simulink model "EnergyHub_V5_inf_buffer"  (R2024b)
settings: Solver=VariableStepAuto  StartTime=0  StopTime=31536000  MaxStep=1  RelTol=1e-3
values from neighbouring files (symbols this model uses):
  BatteryVNom = 51.2    [EdgeCases.m]    (also in MultipleModelTesting.m; setup_V3.m; setup_V5.m)
  ElectrolyserBoP = 80    [EdgeCases.m]    (also in setup_V3.m; setup_V5.m)
  ElectrolyserHoldTime = 25 * 60    (= 1500)    [EdgeCases.m]    (also in setup_V3.m; setup_V5.m)
  ElectrolyserHyFlow = 510    [EdgeCases.m]    (also in setup_V3.m; setup_V5.m)
  ElectrolyserPower = 2450    [EdgeCases.m]    (also in setup_V3.m = 2450/2:2450/2:2450*1.5; setup_V5.m)
  ElectrolyserRampDownTime = 30 * 60    (= 1800)    [EdgeCases.m]    (also in setup_V3.m; setup_V5.m)
  ElectrolyserRampUpTime = 10 * 60    (= 600)    [EdgeCases.m]    (also in setup_V3.m; setup_V5.m)
  ElectrolyserWarming = 260    [EdgeCases.m]    (also in setup_V3.m; setup_V5.m)
  ElectrolyserWarmingTime = 12 * 60    (= 720)    [EdgeCases.m]    (also in setup_V3.m; setup_V5.m)
  EMSElecStartHr = 14    [EdgeCases.m]    (also in setup_V3.m = 12:0.5:15; setup_V5.m)
  EMSElecStartSoC = 70    [EdgeCases.m]    (also in setup_V3.m = 70:5:80; setup_V5.m)
  EMSElecStopSoC = 65    [EdgeCases.m]    (also in setup_V3.m = 50:5:65; setup_V5.m)
  EMSFCSoCThresholds = [140, 150, 160, 170, 180]    [EdgeCases.m]    (also in setup_V3.m = [13, 14, 15, 16, 17]; setup_V5.m)
  EMSFCStartSoC = 15    [EdgeCases.m]    (also in MultipleModelTesting.m; setup_V3.m = 25; setup_V5.m)
  EMSFCStopSoC = 70    [EdgeCases.m]    (also in MultipleModelTesting.m; setup_V3.m = 90; setup_V5.m)
  EMSFCTimeThresholds = [113, 114, 115, 116, 117]    [EdgeCases.m]    (also in setup_V3.m = [40, 50, 60, 70, 80]; setup_V5.m)
  FuelCellAirBlower = 6.4*33.9    (= 216.96)    [EdgeCases.m]    (also in setup_V3.m; setup_V5.m)
  FuelCellBoP = 155    [EdgeCases.m]    (also in setup_V3.m; setup_V5.m)
  FuelCellHyFlow = 24    [EdgeCases.m]    (also in setup_V3.m = 31.7333333333; setup_V5.m)
  FuelCellPower = 2380    [EdgeCases.m]    (also in setup_V3.m = 1.2e3:300:1.8e3; setup_V5.m)
  FuelCellRampDown = 60    [EdgeCases.m]    (also in setup_V3.m; setup_V5.m)
  FuelCellRampTime1 = 40    [EdgeCases.m]    (also in setup_V3.m; setup_V5.m)
  FuelCellRampTime2 = 18*60    (= 1080)    [EdgeCases.m]    (also in setup_V3.m; setup_V5.m)
  FuelCellStartPower = 580    [EdgeCases.m]    (also in setup_V3.m; setup_V5.m)
  GridExtra = 0    [EdgeCases.m]    (also in setup_V3.m; setup_V5.m = 50)
  HydrogenCapacity = 70    [EdgeCases.m]    (also in setup_V3.m = 48; setup_V5.m)
  MinSoCGrid = EMSFCStartSoC-5    (= 10)    [EdgeCases.m]    (also in MultipleModelTesting.m; setup_V5.m)
  SolarPanels = 21    [EdgeCases.m]    (also in MultipleModelTesting.m = 12; setup_V3.m = 12:3:18; setup_V5.m = 18)
  SummerBase = 80    [EdgeCases.m]    (also in setup_V3.m; setup_V5.m)
  WinterBase = 235    [EdgeCases.m]    (also in setup_V3.m; setup_V5.m)
undefined symbols (not defined in the file or in its folder): Ion, Lithium
libraries: spsACVoltageSourceLib x3, spsBatteryLib x1, spsControlledCurrentSourceLib x1, sps_lib x1, simulink x1, spsGroundLib x1, spsPower3phInstantaneousLib x1, spsThreePhaseDynamicLoadLib x1, spsThreePhaseVIMeasurementLib x1
(part 2 of 2)

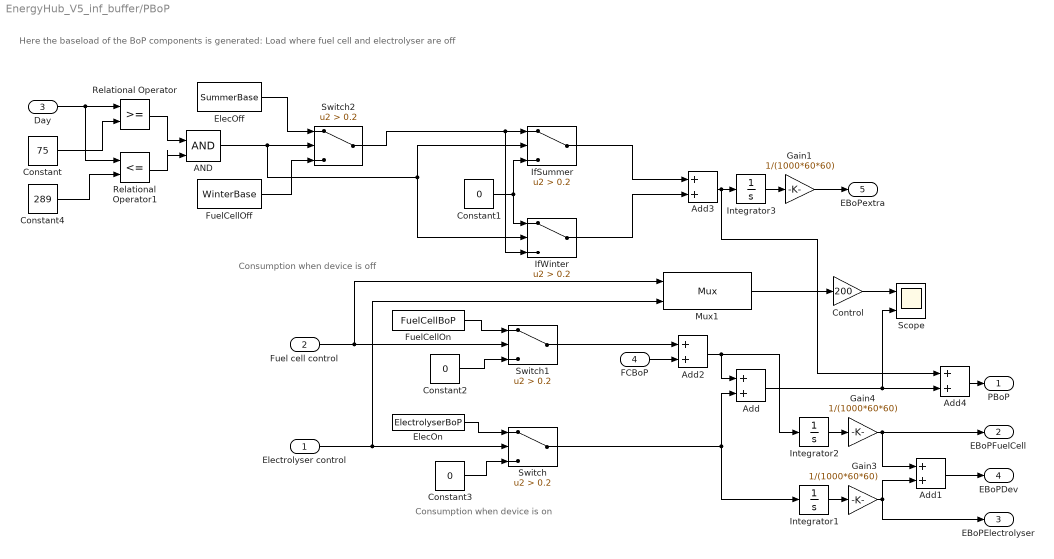
== system EnergyHub_V5_inf_buffer/PBoP ==
  note: Consumption when device is off
  note: Here the baseload of the
      | BoP components is generated:
      | Load where fuel cell and electrolyser are off
  note: Consumption when device is on
  Electrolyser control : Inport
  Fuel cell control : Inport  Port=2
  Day : Inport  Port=3
  FCBoP : Inport  Port=4
  AND : Logic  IconShape=distinctive  AllPortsSameDT=off  OutDataTypeStr=boolean
  Add{,1..4} (5 alike) : Sum
  Constant : Constant  Value=75
  Constant1 : Constant  Value=0
  Constant2 : Constant  Value=0
  Constant3 : Constant  Value=0
  Constant4 : Constant  Value=289
  Control : Gain  Gain=200
  ElecOff : Constant  Value=SummerBase
  ElecOn : Constant  Value=ElectrolyserBoP
  FuelCellOff : Constant  Value=WinterBase
  FuelCellOn : Constant  Value=FuelCellBoP
  Gain1 : Gain  Gain=1/(1000*60*60)
  Gain3 : Gain  Gain=1/(1000*60*60)
  Gain4 : Gain  Gain=1/(1000*60*60)
  IfSummer : Switch  Criteria=u2 > Threshold  Threshold=0.2  SaturateOnIntegerOverflow=off  InputSameDT=off
  IfWinter : Switch  Criteria=u2 > Threshold  Threshold=0.2  SaturateOnIntegerOverflow=off  InputSameDT=off
  Integrator1 : Integrator
  Integrator2 : Integrator
  Integrator3 : Integrator
  Mux1 : Mux  Inputs=2
      settings: DisplayOption=signals
  Relational Operator : RelationalOperator  OutDataTypeStr=boolean  RndMeth=Simplest  InputSameDT=off
  Relational Operator1 : RelationalOperator  Operator=<=  OutDataTypeStr=boolean  RndMeth=Simplest  InputSameDT=off
  Scope : Scope  NumInputPorts=2
  Switch : Switch  Criteria=u2 > Threshold  Threshold=0.2  SaturateOnIntegerOverflow=off  InputSameDT=off
  Switch1 : Switch  Criteria=u2 > Threshold  Threshold=0.2  SaturateOnIntegerOverflow=off  InputSameDT=off
  Switch2 : Switch  Criteria=u2 > Threshold  Threshold=0.2  SaturateOnIntegerOverflow=off  InputSameDT=off
  PBoP : Outport
  EBoPFuelCell : Outport  Port=2
  EBoPElectrolyser : Outport  Port=3
  EBoPDev : Outport  Port=4
  EBoPextra : Outport  Port=5
  wires:
  Switch/1 -> Add/2, Integrator1/1
  Add/1 -> Add4/2, Scope/2
  Add1/1 -> EBoPDev/1
  Gain3/1 -> Add1/2, EBoPElectrolyser/1
  Integrator1/1 -> Gain3/1
  Gain4/1 -> Add1/1, EBoPFuelCell/1
  Integrator2/1 -> Gain4/1
  ElecOn/1 -> Switch/1
  Electrolyser control/1 -> Mux1/2, Switch/2
  Fuel cell control/1 -> Mux1/1, Switch1/2
  FuelCellOn/1 -> Switch1/1
  Day/1 -> Relational Operator1/1, Relational Operator/1
  Constant/1 -> Relational Operator/2
  Constant4/1 -> Relational Operator1/2
  Relational Operator/1 -> AND/1
  Relational Operator1/1 -> AND/2
  AND/1 -> IfSummer/2, IfWinter/2, Switch2/2
  ElecOff/1 -> Switch2/1
  FuelCellOff/1 -> Switch2/3
  Switch2/1 -> IfWinter/3, IfSummer/1
  Constant1/1 -> IfWinter/1, IfSummer/3
  Control/1 -> Scope/1
  Mux1/1 -> Control/1
  Switch1/1 -> Add2/1
  FCBoP/1 -> Add2/2
  Add2/1 -> Add/1, Integrator2/1
  Constant2/1 -> Switch1/3
  Constant3/1 -> Switch/3
  IfSummer/1 -> Add3/1
  IfWinter/1 -> Add3/2
  Add3/1 -> Add4/1, Integrator3/1
  Integrator3/1 -> Gain1/1
  Gain1/1 -> EBoPextra/1
  Add4/1 -> PBoP/1

== system EnergyHub_V5_inf_buffer/PV generation ==
  From Workspace1 : FromWorkspace  VariableName=GTIdays  SampleTime=60  Interpolate=off  OutputAfterFinalValue=Setting to zero
  Gain : Gain  Gain=1/(1000*60*60)
  Integrator : Integrator
  Match Hours : TransportDelay  DelayTime=3600  BufferSize=5120
  eff : Gain  Gain=0.203
  m2 : Gain  Gain=SolarPanels*1.134*1.762
  PVPower : Outport
  PVEnergy : Outport  Port=2
  wires:
  Integrator/1 -> Gain/1
  Gain/1 -> PVEnergy/1
  m2/1 -> eff/1
  eff/1 -> Integrator/1, PVPower/1
  From Workspace1/1 -> Match Hours/1
  Match Hours/1 -> m2/1

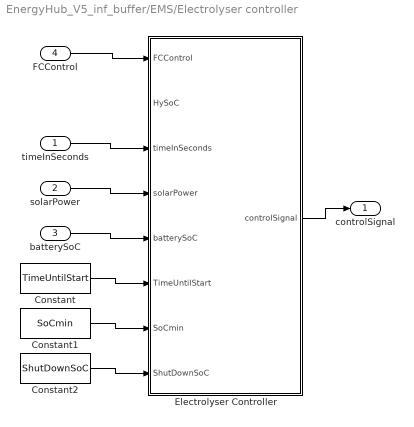
== system EnergyHub_V5_inf_buffer/EMS/Electrolyser controller ==
  timeInSeconds : Inport
  solarPower : Inport  Port=2
  batterySoC : Inport  Port=3
  FCControl : Inport  Port=4
  Constant : Constant  Value=TimeUntilStart
  Constant1 : Constant  Value=SoCmin
  Constant2 : Constant  Value=ShutDownSoC
  Electrolyser Controller : MATLAB Function  TreatAsAtomicUnit=on
  controlSignal : Outport
  wires:
  Electrolyser Controller/1(controlSignal) -> controlSignal/1
  batterySoC/1 -> Electrolyser Controller/5(batterySoC)
  timeInSeconds/1 -> Electrolyser Controller/3(timeInSeconds)
  solarPower/1 -> Electrolyser Controller/4(solarPower)
  Constant/1 -> Electrolyser Controller/6(TimeUntilStart)
  Constant1/1 -> Electrolyser Controller/7(SoCmin)
  Constant2/1 -> Electrolyser Controller/8(ShutDownSoC)
  FCControl/1 -> Electrolyser Controller/1(FCControl)

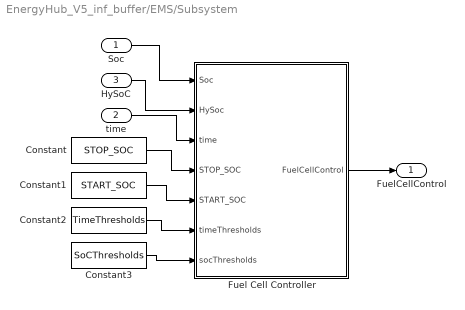
== system EnergyHub_V5_inf_buffer/EMS/Subsystem ==
  Soc : Inport
  time : Inport  Port=2
  HySoC : Inport  Port=3
  Constant : Constant  Value=STOP_SOC
  Constant1 : Constant  Value=START_SOC
  Constant2 : Constant  Value=TimeThresholds
  Constant3 : Constant  Value=SoCThresholds
  Fuel Cell Controller : MATLAB Function  TreatAsAtomicUnit=on
  FuelCellControl : Outport
  wires:
  Soc/1 -> Fuel Cell Controller/1(Soc)
  Fuel Cell Controller/1(FuelCellControl) -> FuelCellControl/1
  time/1 -> Fuel Cell Controller/3(time)
  Constant/1 -> Fuel Cell Controller/4(STOP_SOC)
  Constant1/1 -> Fuel Cell Controller/5(START_SOC)
  Constant3/1 -> Fuel Cell Controller/7(socThresholds)
  Constant2/1 -> Fuel Cell Controller/6(timeThresholds)
  HySoC/1 -> Fuel Cell Controller/2(HySoc)

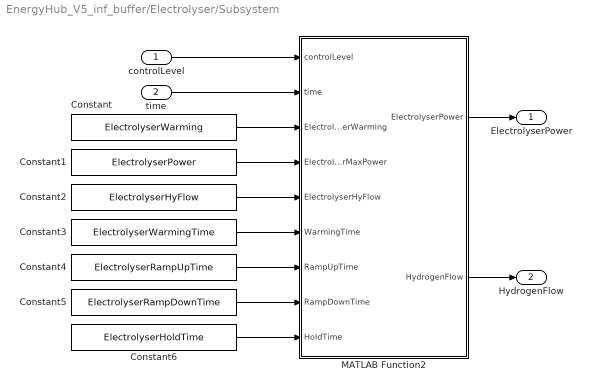
== system EnergyHub_V5_inf_buffer/Electrolyser/Subsystem ==
  controlLevel : Inport
  time : Inport  Port=2
  Constant : Constant  Value=ElectrolyserWarming
  Constant1 : Constant  Value=ElectrolyserPower
  Constant2 : Constant  Value=ElectrolyserHyFlow
  Constant3 : Constant  Value=ElectrolyserWarmingTime
  Constant4 : Constant  Value=ElectrolyserRampUpTime
  Constant5 : Constant  Value=ElectrolyserRampDownTime
  Constant6 : Constant  Value=ElectrolyserHoldTime
  MATLAB Function2 : MATLAB Function  TreatAsAtomicUnit=on
  ElectrolyserPower : Outport
  HydrogenFlow : Outport  Port=2
  wires:
  MATLAB Function2/2(HydrogenFlow) -> HydrogenFlow/1
  MATLAB Function2/1(ElectrolyserPower) -> ElectrolyserPower/1
  controlLevel/1 -> MATLAB Function2/1(controlLevel)
  time/1 -> MATLAB Function2/2(time)
  Constant/1 -> MATLAB Function2/3(ElectrolyserWarming)
  Constant1/1 -> MATLAB Function2/4(ElectrolyserMaxPower)
  Constant2/1 -> MATLAB Function2/5(ElectrolyserHyFlow)
  Constant3/1 -> MATLAB Function2/6(WarmingTime)
  Constant4/1 -> MATLAB Function2/7(RampUpTime)
  Constant5/1 -> MATLAB Function2/8(RampDownTime)
  Constant6/1 -> MATLAB Function2/9(HoldTime)

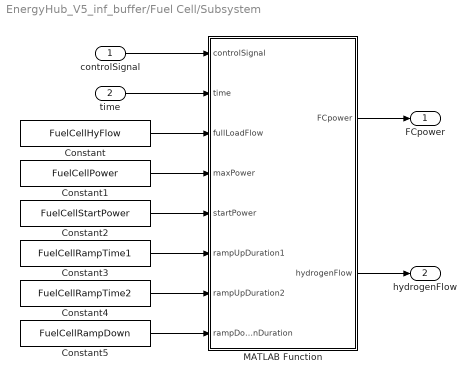
== system EnergyHub_V5_inf_buffer/Fuel Cell/Subsystem ==
  controlSignal : Inport
  time : Inport  Port=2
  Constant : Constant  Value=FuelCellHyFlow
  Constant1 : Constant  Value=FuelCellPower
  Constant2 : Constant  Value=FuelCellStartPower
  Constant3 : Constant  Value=FuelCellRampTime1
  Constant4 : Constant  Value=FuelCellRampTime2
  Constant5 : Constant  Value=FuelCellRampDown
  MATLAB Function : MATLAB Function  TreatAsAtomicUnit=on
  FCpower : Outport
  hydrogenFlow : Outport  Port=2
  wires:
  MATLAB Function/2(hydrogenFlow) -> hydrogenFlow/1
  controlSignal/1 -> MATLAB Function/1(controlSignal)
  MATLAB Function/1(FCpower) -> FCpower/1
  time/1 -> MATLAB Function/2(time)
  Constant/1 -> MATLAB Function/3(fullLoadFlow)
  Constant2/1 -> MATLAB Function/5(startPower)
  Constant1/1 -> MATLAB Function/4(maxPower)
  Constant3/1 -> MATLAB Function/6(rampUpDuration1)
  Constant4/1 -> MATLAB Function/7(rampUpDuration2)
  Constant5/1 -> MATLAB Function/8(rampDownDuration)

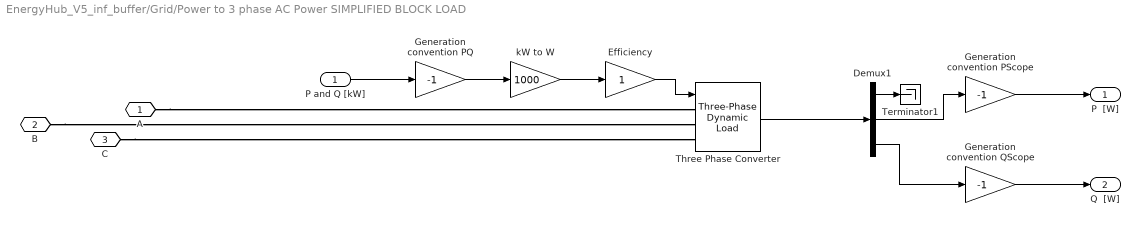
== system EnergyHub_V5_inf_buffer/Grid/Power to 3 phase AC Power SIMPLIFIED BLOCK LOAD ==
  P and Q [kW] : Inport
  Demux1 : Demux  Outputs=3
      settings: DisplayOption=none
  Efficiency : Gain
  Generation convention PQ : Gain  Gain=-1
  Generation convention PScope : Gain  Gain=-1
  Generation convention QScope : Gain  Gain=-1
  Terminator1 : Terminator
  Three Phase Converter : spsThreePhaseDynamicLoadLib/Three-Phase Dynamic Load  NominalVoltage=[ 400 50 ]  ActiveReactivePowers=[50e+003 0]  PositiveSequence=[0.98441 -1.41063]  ExternalControl=on  NpNq="[1  1]"  TimeConstants="[0  0  0  0]"  MinimumVoltage=0.7  Tfilter=1e-4  LoadFlowParameters=[4 50000000 0 0 25000000]
  kW to W : Gain  Gain=1000
  A : PMIOPort  Side=Left
  B : PMIOPort  Port=2  Side=Left
  C : PMIOPort  Port=3  Side=Left
  "P  [W] " : Outport
  "Q  [W] " : Outport  Port=2
  wires:
  Demux1/1 -> Terminator1/1
  Efficiency/1 -> Three Phase Converter/1
  kW to W/1 -> Efficiency/1
  Generation convention PQ/1 -> kW to W/1
  P and Q [kW]/1 -> Generation convention PQ/1
  Generation convention PScope/1 -> "P  [W] "/1
  Demux1/2 -> Generation convention PScope/1
  Demux1/3 -> Generation convention QScope/1
  Generation convention QScope/1 -> "Q  [W] "/1
  Three Phase Converter/1 -> Demux1/1
  connections:
  A/RConn1 -- Three Phase Converter/LConn1
  C/RConn1 -- Three Phase Converter/LConn3
  B/RConn1 -- Three Phase Converter/LConn2

== matlab function EnergyHub_V5_inf_buffer/Electrolyser/Subsystem/MATLAB Function2 ==
  settings: updateMethod=DISCRETE
  data: controlLevel input; ElectrolyserPower output; time input; HydrogenFlow output; ElectrolyserWarming input; ElectrolyserMaxPower input; ElectrolyserHyFlow input; WarmingTime input; RampUpTime input; RampDownTime input; HoldTime input
function [ElectrolyserPower, HydrogenFlow] = Electrolyser(controlLevel, time, ElectrolyserWarming, ElectrolyserMaxPower, ElectrolyserHyFlow, WarmingTime, RampUpTime, RampDownTime, HoldTime)
    % Inputs:
    % controlLevel (double): Control level between 0.6 and 1.0, 0 means off, and values between 0.6 and 1.0 represent the operational level
    % time (double): Simulation time in seconds
    
    % Outputs:
    % ElectrolyserPower (double): Power consumed by the electrolyser
    % HydrogenFlow (double): Hydrogen flow rate
    
    % Constants
    %ElectrolyserWarming = 260;  % [W] Electrolyser Warming Power Consumption
    %ElectrolyserPower = 2450;   % [W] Electrolyser Max Power Consumption
    %ElectrolyserHyFlow = 510;
    %WarmingTime = 12 * 60; % 12 minutes in seconds
    %RampUpTime = 10 * 60; % 10 minutes in seconds
    %RampDownTime = 30 * 60;
    RampDownStartPower = 0.6 * ElectrolyserMaxPower;
    RampDownStartHy = 0.6 * ElectrolyserHyFlow;
    %HoldTime = 25 * 60;         % Time before electrolyser actually turns off after off signal

    % Logic for output control
    persistent startTime isRampActive stopTime isRampingDown currentPower currentHydrogen;

    % Initialize persistent variables
    if isempty(startTime) || isempty(isRampActive) || isempty(isRampingDown) || isempty(stopTime)
        startTime = NaN;
        stopTime = NaN;
        isRampActive = false;
        isRampingDown = false;
        currentPower = 0;
        currentHydrogen = 0;
    end

    % Default outputs
    ElectrolyserPower = 0;
    HydrogenFlow = 0;

    % Initialize target variables
    targetPower = 0;
    targetHydrogen = 0;

    % If the control level is nonzero (system is on)
    if controlLevel > 0
        % If the system has not started before, record the start time
        if isnan(startTime)
            startTime = time;
            isRampActive = false; % Start with constant output
        end

        % If the system has been running for 12 minutes, start ramping
        if (time - startTime) >= WarmingTime && ~isRampActive
            isRampActive = true; % Start ramping after 12 minutes
        end

        % If the system is ramping
        if isRampActive
            % Calculate elapsed time for ramp-up
            rampElapsedTime = time - startTime - WarmingTime;

            % If the ramping time has not yet completed, linearly ramp from 260 to 2450
            if rampElapsedTime <= RampUpTime
                targetPower = ElectrolyserWarming + (ElectrolyserMaxPower - ElectrolyserWarming) * (rampElapsedTime / RampUpTime) * controlLevel;
                targetHydrogen = 0 + (ElectrolyserHyFlow - 0) * (rampElapsedTime / RampUpTime) * controlLevel;
            else
                % Once ramp-up is complete, keep the output at the final ramp values scaled by controlLevel
                targetPower = ElectrolyserMaxPower * controlLevel;
                targetHydrogen = ElectrolyserHyFlow * controlLevel;
            end
        else
            % If still within the first 12 minutes, output the constant value scaled by controlLevel
            targetPower = ElectrolyserWarming; %* controlLevel;
            targetHydrogen = 0; % Assume no hydrogen flow during the constant phase
        end
    else
        % Check if the system was previously on before ramping down
        if ~isnan(startTime)
            if isnan(stopTime)
                stopTime = time; % Record time when system turned off
                isRampingDown = true;
            end

            rampDownElapsedTime = time - stopTime;

            if isRampingDown
                if rampDownElapsedTime <= RampDownTime
                    % Ramp down power from previous state
                    targetPower = currentPower - (currentPower - RampDownStartPower * controlLevel) * (rampDownElapsedTime / RampDownTime);
                    targetHydrogen = currentHydrogen - (currentHydrogen - RampDownStartHy * controlLevel) * (rampDownElapsedTime / RampDownTime);
                elseif rampDownElapsedTime <= (RampDownTime + HoldTime)
                    % Hold at 60% power
                    targetPower = RampDownStartPower * controlLevel;
                    targetHydrogen = RampDownStartHy * controlLevel;
                else
                    % Fully shut down
                    targetPower = 0;
                    targetHydrogen = 0;
                    isRampingDown = false; % Stop ramp-down process
                    startTime = NaN; % Fully reset system
                    stopTime = NaN;
                    isRampActive = false;
                end
            end
        else
            % If the system was never on, ensure it stays off
            targetPower = 0;
            targetHydrogen = 0;
        end
    end

    % Smooth transition to target values
    rampRate = 50; % Rate of power change per time step
    if currentPower < targetPower
        currentPower = min(currentPower + rampRate, targetPower);
    elseif currentPower > targetPower
        currentPower = max(currentPower - rampRate, targetPower);
    end

    if currentHydrogen < targetHydrogen
        currentHydrogen = min(currentHydrogen + rampRate, targetHydrogen);
    elseif currentHydrogen > targetHydrogen
        currentHydrogen = max(currentHydrogen - rampRate, targetHydrogen);
    end

    ElectrolyserPower = currentPower;
    HydrogenFlow = currentHydrogen;
end

== matlab function EnergyHub_V5_inf_buffer/EMS/Subsystem/Fuel Cell Controller ==
  settings: updateMethod=DISCRETE
  data: Soc input; HySoc input; time input; FuelCellControl output; STOP_SOC input; START_SOC input; timeThresholds input; socThresholds input
function FuelCellControl = fuelCellControl(Soc, HySoc, time,STOP_SOC, START_SOC, timeThresholds, socThresholds)
    % Inputs:
    % Soc: Battery State of Charge (SoC) in percentage (0-100)
    % time: Current simulation time in seconds
    
    % Outputs:
    % FuelCellControl: on (1) or off (0)
    
    % Constants
    % STOP_SOC, Stop fuel cell if SoC > 90%
    % START_SOC, Start fuel cell if SoC < 25%
    
    % Define SoC thresholds for different times of day
    % timeThresholds, 13:00, 14:00, 15:00, 16:00, 17:00 (in hours)
    % socThresholds, 40, 50, 60, 70, 80: Corresponding SoC thresholds
    
    % Convert time from seconds to hours
    timeInHours = mod(time / 3600, 24);
    
    % Persistent variable to track whether the fuel cell remains on
    persistent hasRunToday;  % Tracks whether the electrolyzer has run today
    persistent Remain;
    persistent lastDay;      % Tracks the last day for resetting logic
    persistent firstSimulatedDay;

    
    if isempty(Remain)
        Remain = 0;         % Initialize to off
    end
    
    if isempty(hasRunToday)
       hasRunToday = true;      % Initially, the electrolyzer has not run today
       lastDay = -2;            % Initialize to an invalid day number
    end
    % Convert time from seconds to hours and extract the hour of the day
    currentDay = floor(time / 86400);      % Day number (0, 1, 2, ...)
    secondsInDay = 86400;
    dayOfYear = floor(time / secondsInDay) + 1; % Day of the year (1 to 365/366)

    OperationalDaysStop = 75;       % Last day of normal fuel cell operation
    OperationalDaysStart = 289;     % First day of normal fuel cell operation

    % Check if the day has changed (midnight reset)
    if currentDay ~= lastDay
       hasRunToday = false;
       lastDay = currentDay; 
       disp(sprintf('New day: %d', int32(currentDay)));   % Prints the current day in the console to track progression
    end

    if isempty(firstSimulatedDay)
        firstSimulatedDay = floor(time / 86400);
    end

    % Ensure fuel cell is off only during the first night of the first simulated day
    if (currentDay == firstSimulatedDay) && (timeInHours < 13)
        FuelCellControl = 0;
        return;
    end

    FuelCellControl = 0; % Initially off


    % Logic to control the fuel cell
  
  
    if Soc < START_SOC
        FuelCellControl = 1;
        Remain = 1;
    elseif Soc > STOP_SOC
        FuelCellControl = 0;
        Remain = 0;
    elseif (Soc >= START_SOC && Soc <= STOP_SOC && currentDay ~= 0)
        if Remain == 1
            FuelCellControl = 1;                % Keep the fuel cell on
            hasRunToday = true;
        else
            for i = 1:length(timeThresholds)    % Check the conditions of the 
                if (timeInHours >= timeThresholds(i) && (i == length(timeThresholds) || timeInHours < timeThresholds(i+1))) && Soc < socThresholds(i) && ~hasRunToday && (dayOfYear <= OperationalDaysStop|| dayOfYear >= OperationalDaysStart )
                    FuelCellControl = 1;        % Fuel cell on
                    hasRunToday = true;
                    Remain = 1;                 % Update Remain to keep it on
                    break;
                end
            end
        end
    end
end

== matlab function EnergyHub_V5_inf_buffer/EMS/Electrolyser controller/Electrolyser Controller ==
  settings: updateMethod=DISCRETE
  data: FCControl input; HySoC input; timeInSeconds input; controlSignal output; solarPower input; batterySoC input; TimeUntilStart input; SoCmin input; ShutDownSoC input
function controlSignal = electrolyzerControl(FCControl, HySoC, timeInSeconds, solarPower, batterySoC, TimeUntilStart, SoCmin, ShutDownSoC)
    % Inputs:
    % - timeInSeconds: Current simulation time in seconds, to determine day
    % - solarPower: Solar power available in W
    % - batterySoC: Battery state of charge in % (0 to 100)
   
    % Output:
    % - controlSignal: 0 = OFF, 0.6 to 1.0 = ON

    % Persistent variables to store state across time steps
    persistent hasRunToday;         % Tracks whether the electrolyzer has run today
    persistent FCHasRunToday;       % Tracks whether the fuel cell has
    persistent FCHasRunYesterday;   % Tracks whether the fuel cell has run yesterday
    persistent lastDay;             % Tracks the last day for resetting logic
    persistent isElectrolyzerOn;    % Tracks whether the electrolyzer is on
    persistent currentControlLevel; % Tracks the current control level

    % Initialize persistent variables
    if isempty(hasRunToday)
        hasRunToday = false;     % Initially, the electrolyzer has not run today
        FCHasRunToday = false;   % Initially, the fuel cell has not run today
        FCHasRunYesterday = false; % Initially, the fuel cell has not run yesterday

        lastDay = -1;            % Initialize to an invalid day number
        isElectrolyzerOn = false; % Initially OFF
        
        currentControlLevel = 0;  % Initially OFF
    end

    % Convert time from seconds to hours and extract the hour of the day
    timeInHours = mod(timeInSeconds, 86400) / 3600; % Hours within a single day
    currentDay = floor(timeInSeconds / 86400);      % Day number (0, 1, 2, ...)

    % Check if the day has changed (midnight reset)
    if currentDay ~= lastDay
        hasRunToday = false;     % Reset for the new day
        FCHasRunYesterday = FCHasRunToday; % Yesterday's FC activity is stored
        FCHasRunToday = false;   % Reset FC run tracking
        lastDay = currentDay;    % Update the lastDay variable
    end

    if FCControl > 0
        FCHasRunToday = true;
    end


    % ON condition: Turn ON the electrolyzer if all conditions are met
    if ~isElectrolyzerOn && ~hasRunToday && batterySoC > SoCmin && solarPower > 1000 && timeInHours < TimeUntilStart && ~FCHasRunToday && ~FCHasRunYesterday
        isElectrolyzerOn = true;  % Turn ON the electrolyzer
        hasRunToday = true;       % Mark as run for the day
    end

    % OFF condition: Turn OFF the electrolyzer if any OFF condition is met
    if isElectrolyzerOn && (batterySoC < ShutDownSoC || solarPower < 50)
        isElectrolyzerOn = false; % electrolyser is shut off
    end

    % Set control signal based on battery SoC when ON
    if isElectrolyzerOn
        targetControlLevel = 0.6 + (batterySoC - SoCmin) / 10  * 0.4; % Scale between 0.6 and 1.0 for SoC ranges
        targetControlLevel = max(0.6, min(targetControlLevel, 1.0));  % Saturate output
        
        % Ramp-up behavior
        rampRate = 0.05; % Rate at which control level increases per step
        if currentControlLevel < targetControlLevel
            currentControlLevel = min(currentControlLevel + rampRate, targetControlLevel);
        elseif currentControlLevel > targetControlLevel
            currentControlLevel = max(currentControlLevel - rampRate, targetControlLevel);
        end
    else
        currentControlLevel = 0; % OFF state
    end
    controlSignal = currentControlLevel;
end

== matlab function EnergyHub_V5_inf_buffer/Fuel Cell/Subsystem/MATLAB Function ==
  settings: updateMethod=DISCRETE
  data: controlSignal input; FCpower output; time input; hydrogenFlow output; fullLoadFlow input; maxPower input; startPower input; rampUpDuration1 input; rampUpDuration2 input; rampDownDuration input
function [FCpower, hydrogenFlow] = fuelCell(controlSignal, time, fullLoadFlow, maxPower, startPower, rampUpDuration1, rampUpDuration2, rampDownDuration)
   % Define the ramp-up and ramp-down parameters
   %rampUpDuration1 = 40; % seconds to ramp from 0W to 500W
   % rampUpDuration2 = 18 * 60; % seconds to ramp from 500W to 1.83kW
   % startPower = 580;
   % maxPower = 1.83e3; % Maximum power in watts (1.83 kW)
    minPower = 0; % Minimum power (0W)
   % fullLoadFlow = 24; % Hydrogen flow rate at full load (NL/min)
   % rampDownDuration = 60; % seconds to ramp down from 1.83kW to 0W

    % Initialize output values
    FCpower = 0;
    hydrogenFlow = 0;

   persistent startTime stopTime isRampActive;
   % Initialize persistent variables
   if isempty(startTime) || isempty(isRampActive) || isempty(stopTime)
       startTime = NaN;
       stopTime = NaN;
       isRampActive = false;
   end
  
    % Check control signal (assuming high is 1 and low is 0)
    if controlSignal == 1       
        if isnan(startTime)
           startTime = time;
           isRampActive = false; % Start with constant output
        end

        rampElapsedTime = time - startTime;

        % Fuel cell is ON, calculate output power and hydrogen flow rate
        if rampElapsedTime <= rampUpDuration1
            % Ramp-up from 0W to 500W in 40 seconds
            FCpower = (startPower / rampUpDuration1) * rampElapsedTime;
        elseif rampElapsedTime <= (rampUpDuration1 + rampUpDuration2)
            % Ramp-up from 500W to 1.83kW in 15 minutes (900 seconds)
            timeInRampUp2 = rampElapsedTime - rampUpDuration1;
            FCpower = startPower + ((maxPower - startPower) / rampUpDuration2) * timeInRampUp2;
        elseif rampElapsedTime > (rampUpDuration1 + rampUpDuration2)
            % Keep the power at 1.83 kW
            FCpower = maxPower;
        end
        
        % Hydrogen flow rate follows the same pattern as power output
        hydrogenFlow = (fullLoadFlow / maxPower) * FCpower;
        
    elseif controlSignal == 0
        % Fuel cell is OFF, calculate ramp-down behavior
        if time <= rampDownDuration
            % Ramp-down from 1.83 kW to 0W in 1 minute
            FCpower = maxPower * (1 - (time / rampDownDuration));
        else
            % Fuel cell is completely off
            FCpower = 0;
            hydrogenFlow = 0;
            startTime = NaN;
        end
    end
end

== matlab function EnergyHub_V5_inf_buffer/Electrolyser/MATLAB Function1 ==
  settings: updateMethod=DISCRETE
  data: startSystem input; ElectrolyserPower output; time input; HydrogenFlow output
function [ElectrolyserPower, HydrogenFlow] = Electrolyser(startSystem, time)
    % Inputs:
    % startSystem (boolean): Indicates whether the system is allowed to start
    % time (double): Simulation time in seconds
    
    % Outputs:
    % ElectrolyserPower (double): Power consumed by the electrolyser
    % HydrogenFlow (double): Hydrogen flow rate
    
    % Constants
    CONSTANT_OUTPUT = 260;
    RAMP_OUTPUT_END = 2450;
    RAMP_OUTPUT_END2 = 510;
    CONSTANT_TIME = 12 * 60; % 12 minutes in seconds
    RAMP_TIME = 10 * 60; % 10 minutes in seconds
    RAMP_DOWN_TIME = 30 * 60;
    RAMP_DOWN_START = 0.6*RAMP_OUTPUT_END;
    RAMP_DOWN_START2 = 0.6* RAMP_OUTPUT_END2;
    HOLD_TIME = 25*60;

    % Logic for output control
    persistent startTime isRampActive stopTime isRampingDown;

    % Initialize persistent variables
    if isempty(startTime) || isempty(isRampActive) || isempty(isRampingDown) || isempty(stopTime)
        startTime = NaN;
        stopTime = NaN;
        isRampActive = false;
        isRampingDown = false;
    end

    % Default outputs
    ElectrolyserPower = 0;
    HydrogenFlow = 0;

    % If the system is turned on
    if startSystem
        % If the system has not started before, record the start time
        if isnan(startTime)
            startTime = time;
            isRampActive = false; % Start with constant output
        end

        % If the system has been running for 12 minutes, start ramping
        if (time - startTime) >= CONSTANT_TIME && ~isRampActive
            isRampActive = true; % Start ramping after 12 minutes
        end

        % If the system is ramping
        if isRampActive
            % Calculate elapsed time for ramp-up
            rampElapsedTime = time - startTime - CONSTANT_TIME;

            % If the ramping time has not yet completed, linearly ramp from 260 to 2450
            if rampElapsedTime <= RAMP_TIME
                ElectrolyserPower = CONSTANT_OUTPUT + (RAMP_OUTPUT_END - CONSTANT_OUTPUT) * (rampElapsedTime / RAMP_TIME);
                HydrogenFlow = 0 + (RAMP_OUTPUT_END2 - 0) * (rampElapsedTime / RAMP_TIME);
            else
                % Once ramp-up is complete, keep the output at the final ramp values
                ElectrolyserPower = RAMP_OUTPUT_END;
                HydrogenFlow = RAMP_OUTPUT_END2;
            end
        else
            % If still within the first 12 minutes, output the constant value
            ElectrolyserPower = CONSTANT_OUTPUT;
            HydrogenFlow = 0; % Assume no hydrogen flow during the constant phase
        end
    else
        % Check if the system was previously on before ramping down
        if ~isnan(startTime)
            if isnan(stopTime)
                stopTime = time; % Record time when system turned off
                isRampingDown = true;
            end

            rampDownElapsedTime = time - stopTime;

            if isRampingDown
                if rampDownElapsedTime <= RAMP_DOWN_TIME
                    % Ramp down power from 100% to 60%
                    ElectrolyserPower = RAMP_OUTPUT_END - (RAMP_OUTPUT_END - RAMP_DOWN_START) * (rampDownElapsedTime / RAMP_DOWN_TIME);
                    HydrogenFlow = RAMP_OUTPUT_END2 - (RAMP_OUTPUT_END2 - RAMP_DOWN_START2) * (rampDownElapsedTime / RAMP_DOWN_TIME);
                elseif rampDownElapsedTime <= (RAMP_DOWN_TIME + HOLD_TIME)
                    % Hold at 60% power
                    ElectrolyserPower = RAMP_DOWN_START;
                    HydrogenFlow = RAMP_DOWN_START2;
                else
                    % Fully shut down
                    ElectrolyserPower = 0;
                    HydrogenFlow = 0;
                    isRampingDown = false; % Stop ramp-down process
                    startTime = NaN; % Fully reset system
                    stopTime = NaN;
                    isRampActive = false;
                end
            end
        else
            % If the system was never on, ensure it stays off
            ElectrolyserPower = 0;
            HydrogenFlow = 0;
        end
    end
end

== matlab function EnergyHub_V5_inf_buffer/MATLAB Function ==
  data: time input; day_num output
function day_num = get_day(time)
    % Convert simulation time (seconds) to days
    seconds_per_day = 24*60*60;
    day_num = floor(time / seconds_per_day) + 1;
end
